simulink model "Purdue_Sim_Fast"  (R2018b)
settings: Solver=VariableStepAuto  StartTime=0.0  StopTime=300  RelTol=1e-3
values from neighbouring files (symbols this model uses):
  burn_time = (200000+Impulse_Savings)/Thrust    [One_Run.m]    (also in Purdue_Setup.m = 40; Setup.m = 42; Test_Runs.m = 40; Test_Runs_Arthur_Function.m = 42.7553241067)
  data = [Mass_b Mass_c]    [Boattail.m]    (also in One_Run.m = load('aerodata.csv'); Purdue_Setup.m = load('aerodata.csv'); Setup.m = load('aerodata.csv'); Test_Runs.m = load('aerodata.csv'))
  diameter_ft = diameter / 12    (= 1.5)    [One_Run.m]    (also in Purdue_Setup.m; Setup.m = 0.535416666667; Test_Runs.m; Test_Runs_Arthur_Function.m)
  dry_mass_slugs = dry_mass / 32.2    [One_Run.m]    (also in Purdue_Setup.m = 12.4223602484; Setup.m = 1.28260869565; Test_Runs.m; Test_Runs_Arthur_Function.m)
  m_dot_slugs = m_dot / 32.2    (= 0.585403726708)    [One_Run.m]    (also in Purdue_Setup.m = -0.621118012422; Setup.m = 0.0567139899438; Test_Runs.m = -0.621118012422; Test_Runs_Arthur_Function.m = -0.62217941157)
  wet_mass_slugs = wet_mass / 32.2    (= 40.8444099379)    [One_Run.m]    (also in Purdue_Setup.m = 37.2670807453; Setup.m = 3.66459627329; Test_Runs.m = wet_mass / 32.2; Test_Runs_Arthur_Function.m = wet_mass / 32.2)
undefined symbols (not defined in the file or in its folder): Thurst
libraries: aerolibasang x2, aerolibconvert2 x2, shared6dof x1, aerolibadyn x1, aerolibatmos2 x1, simulink x1, vrlib x1
settings Model: PacingRate=1000  Creator=jbartkie  LastModifiedBy=bartk
settings DebuggingCC: LibraryContextMissingDiagnostic=none  UnderSpecifiedDimensionMsg=warning
settings SFSimCC: SimUseLocalCustomCode=off
settings RTWCC: RTWUseLocalCustomCode=off

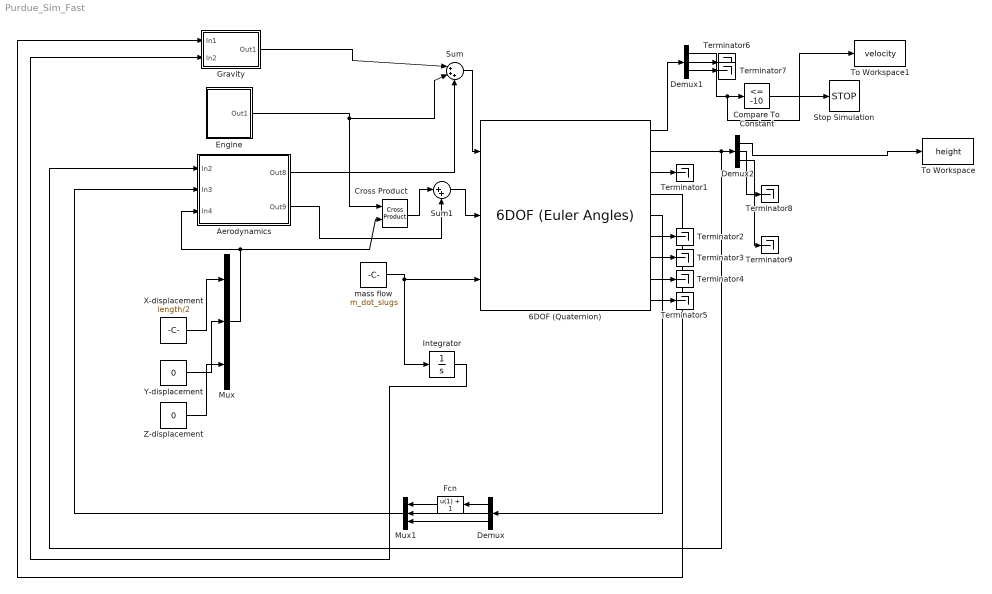
== system Purdue_Sim_Fast ==
  6DOF (Quaternion) : shared6dof/6DOF (Euler Angles)  units=English (Velocity in ft/s)  mtype=Simple Variable  rep=Quaternion  xme_0=[0 0 0]  Vm_0=[0 0 0]  eul_0=[0 0 0]  pm_0=[0 0 0]  mass_0=wet_mass_slugs  mass_e=dry_mass_slugs  mass_f=wet_mass_slugs  inertia=eye(3)  inertia_e=I_wet  inertia_f=I_dry  k_quat=1.0  vre_flag=off  abi_flag=off  aMode=0  xme_statename=''  Vm_statename=''  eul_statename=''  quat_statename=''  pm_statename=''  mass_statename=''
      settings: SourceProductBaseCode=AE
  "Aerodynamics " : Subsystem
  Compare To Constant : simulink/Logic and Bit Operations/Compare To Constant  relop=<=  const=-10  OutDataTypeStr=boolean
  Cross Product : vrlib/Utilities/Cross Product
      settings: SourceProductBaseCode=VR
  Demux : Demux  Outputs=3
  Demux1 : Demux  Outputs=3
  Demux2 : Demux  Outputs=3
  "Engine " : Subsystem
  Fcn : Fcn  Expr=u(1) + 1
  Gravity : Subsystem
  Integrator : Integrator  InitialCondition=wet_mass_slugs  LimitOutput=on  LowerSaturationLimit=dry_mass_slugs
  Mux : Mux  Inputs=3
  Mux1 : Mux  Inputs=3
  Stop Simulation : Stop
  Sum : Sum  Inputs=|+++
  Sum1 : Sum  Inputs=|++
  Terminator{1..9} (9 alike) : Terminator
  To Workspace : ToWorkspace  VariableName=height  SaveFormat=Timeseries  SampleTime=-1
  To Workspace1 : ToWorkspace  VariableName=velocity  SaveFormat=Timeseries  SampleTime=-1
  X-displacement : Constant  Value=length/2
  Y-displacement : Constant  Value=0
  Z-displacement : Constant  Value=0
  mass flow : Constant  Value=m_dot_slugs
  wires:
  Z-displacement/1 -> Mux/3
  X-displacement/1 -> Mux/1
  Y-displacement/1 -> Mux/2
  "Engine "/1(Out1) -> Cross Product/1, Sum/2
  Sum/1 -> 6DOF (Quaternion)/1
  Gravity/1(Out1) -> Sum/1
  Integrator/1 -> Gravity/2(In2)
  mass flow/1 -> Integrator/1, 6DOF (Quaternion)/3
  6DOF (Quaternion)/4 -> Gravity/1(In1)
  Sum1/1 -> 6DOF (Quaternion)/2
  Cross Product/1 -> Sum1/1
  Mux/1 -> Cross Product/2, "Aerodynamics "/3(In4)
  "Aerodynamics "/1(Out8) -> Sum/3
  "Aerodynamics "/2(Out9) -> Sum1/2
  6DOF (Quaternion)/5 -> Demux/1
  Demux/2 -> Mux1/2
  Demux/3 -> Mux1/3
  Demux/1 -> Fcn/1
  Fcn/1 -> Mux1/1
  Mux1/1 -> "Aerodynamics "/2(In3)
  6DOF (Quaternion)/1 -> Demux1/1
  6DOF (Quaternion)/3 -> Terminator1/1
  6DOF (Quaternion)/6 -> Terminator2/1
  6DOF (Quaternion)/7 -> Terminator3/1
  6DOF (Quaternion)/8 -> Terminator4/1
  6DOF (Quaternion)/9 -> Terminator5/1
  6DOF (Quaternion)/2 -> Demux2/1, "Aerodynamics "/1(In2)
  Demux1/1 -> To Workspace1/1, Compare To Constant/1
  Compare To Constant/1 -> Stop Simulation/1
  Demux1/2 -> Terminator6/1
  Demux1/3 -> Terminator7/1
  Demux2/1 -> To Workspace/1
  Demux2/2 -> Terminator8/1
  Demux2/3 -> Terminator9/1

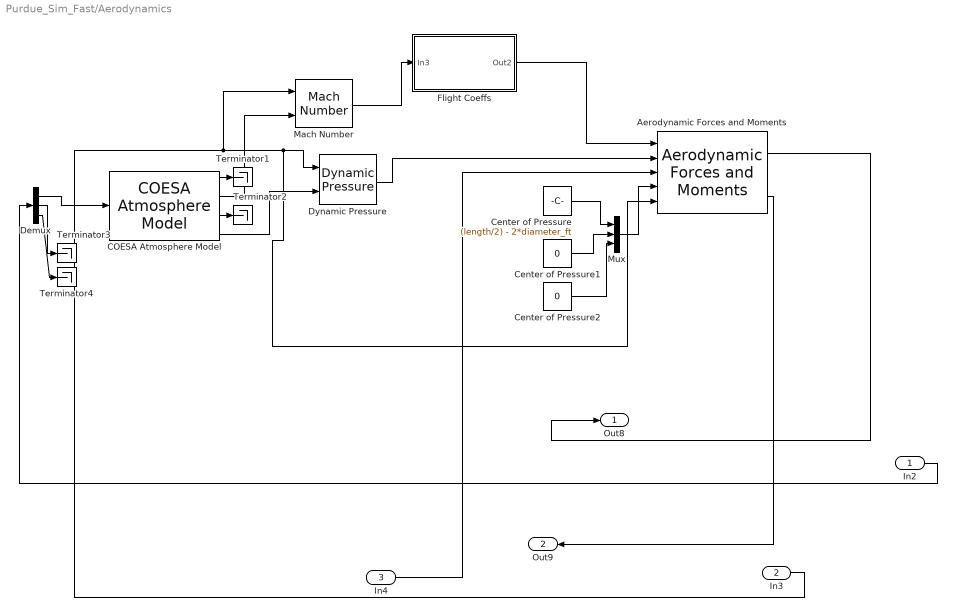
== system Purdue_Sim_Fast/Aerodynamics  ==
  In2 : Inport
  In3 : Inport  Port=2
  In4 : Inport  Port=3
  "Aerodynamic Forces and Moments " : aerolibadyn/Aerodynamic Forces and Moments   inputAxes=Wind  outputForceAxes=Body  outputMomentAxes=Body  S=(diameter_ft/2)^2 * pi  b=diameter_ft  cbar=length
      settings: SourceProductName=Aerospace Blockset
  COESA Atmosphere Model : aerolibatmos2/COESA Atmosphere Model  units=English (Velocity in ft/s)  spec=1976 COESA-extended U.S. Standard Atmosphere  model=Profile  profile_var=High temperature  profile_percent=1%  profile_alt=5 km (16404 ft)  envelope_var=High temperature  envelope_percent=1%  action=Warning
  Center of Pressure : Constant  Value=(length/2) - 2*diameter_ft
  Center of Pressure1 : Constant  Value=0
  Center of Pressure2 : Constant  Value=0
  Demux : Demux  Outputs=3
  Dynamic Pressure : aerolibasang/Dynamic Pressure
  Flight Coeffs : Subsystem
  Mach Number : aerolibasang/Mach Number
      settings: SourceProductName=Aerospace Blockset  SourceProductBaseCode=AE
  Mux : Mux  Inputs=3
  Terminator{1..4} (4 alike) : Terminator
  Out8 : Outport
  Out9 : Outport  Port=2
  wires:
  Dynamic Pressure/1 -> "Aerodynamic Forces and Moments "/2
  Demux/1 -> COESA Atmosphere Model/1
  In2/1 -> Demux/1
  In4/1 -> "Aerodynamic Forces and Moments "/3
  COESA Atmosphere Model/4 -> Dynamic Pressure/2
  COESA Atmosphere Model/2 -> Mach Number/2
  In3/1 -> Mach Number/1, "Aerodynamic Forces and Moments "/5, Dynamic Pressure/1
  "Aerodynamic Forces and Moments "/2 -> Out9/1
  Mach Number/1 -> Flight Coeffs/1(In3)
  Flight Coeffs/1(Out2) -> "Aerodynamic Forces and Moments "/1
  Mux/1 -> "Aerodynamic Forces and Moments "/4
  Center of Pressure/1 -> Mux/1
  Center of Pressure1/1 -> Mux/2
  Center of Pressure2/1 -> Mux/3
  "Aerodynamic Forces and Moments "/1 -> Out8/1
  COESA Atmosphere Model/1 -> Terminator1/1
  COESA Atmosphere Model/3 -> Terminator2/1
  Demux/2 -> Terminator3/1
  Demux/3 -> Terminator4/1

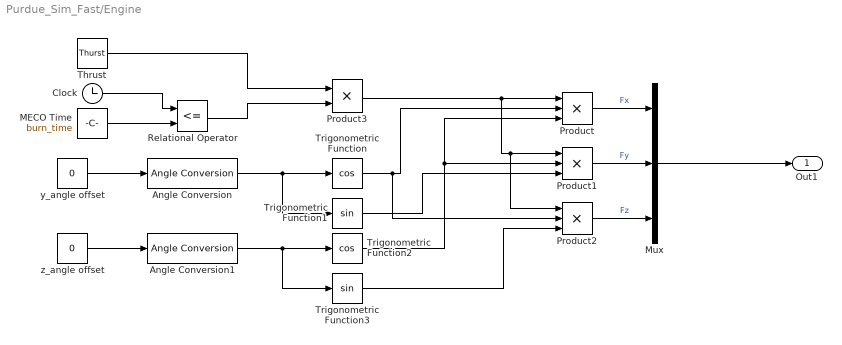
== system Purdue_Sim_Fast/Engine  ==
  Angle Conversion : aerolibconvert2/Angle Conversion  IU=deg  OU=rad
  Angle Conversion1 : aerolibconvert2/Angle Conversion  IU=deg  OU=rad
  Clock : Clock
  MECO Time : Constant  Value=burn_time
  Mux : Mux  Inputs=3
  Product : Product  Inputs=3
  Product1 : Product  Inputs=3
  Product2 : Product  Inputs=3
  Product3 : Product
  Relational Operator : RelationalOperator  Operator=<=  OutDataTypeStr=boolean  RndMeth=Simplest
  Thrust : Constant  Value=Thurst
  Trigonometric Function : Trigonometry  Operator=cos
  Trigonometric Function1 : Trigonometry
  Trigonometric Function2 : Trigonometry  Operator=cos
  Trigonometric Function3 : Trigonometry
  y_angle offset : Constant  Value=0
  z_angle offset : Constant  Value=0
  Out1 : Outport
  wires:
  Angle Conversion/1 -> Trigonometric Function1/1, Trigonometric Function/1
  Angle Conversion1/1 -> Trigonometric Function3/1, Trigonometric Function2/1
  Clock/1 -> Relational Operator/1
  MECO Time/1 -> Relational Operator/2
  Thrust/1 -> Product3/1
  Relational Operator/1 -> Product3/2
  Product/1 -> Mux/1  "Fx"
  Product1/1 -> Mux/2  "Fy"
  Product2/1 -> Mux/3  "Fz"
  Mux/1 -> Out1/1
  Product3/1 -> Product2/1, Product1/1, Product/1
  Trigonometric Function2/1 -> Product1/2, Product/3
  Trigonometric Function/1 -> Product2/2, Product/2
  Trigonometric Function1/1 -> Product1/3
  Trigonometric Function3/1 -> Product2/3
  y_angle offset/1 -> Angle Conversion/1
  z_angle offset/1 -> Angle Conversion1/1

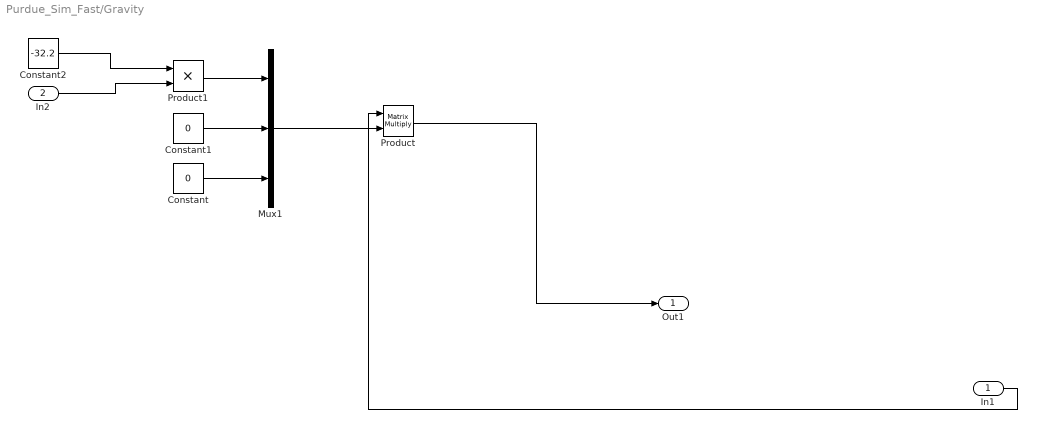
== system Purdue_Sim_Fast/Gravity ==
  In1 : Inport
  In2 : Inport  Port=2
  Constant : Constant  Value=0
  Constant1 : Constant  Value=0
  Constant2 : Constant  Value=-32.2
  Mux1 : Mux  Inputs=3
  Product : Product  Multiplication=Matrix(*)
  Product1 : Product
  Out1 : Outport
  wires:
  Mux1/1 -> Product/2
  Product/1 -> Out1/1
  In1/1 -> Product/1
  Constant1/1 -> Mux1/2
  Constant2/1 -> Product1/1
  In2/1 -> Product1/2
  Product1/1 -> Mux1/1
  Constant/1 -> Mux1/3

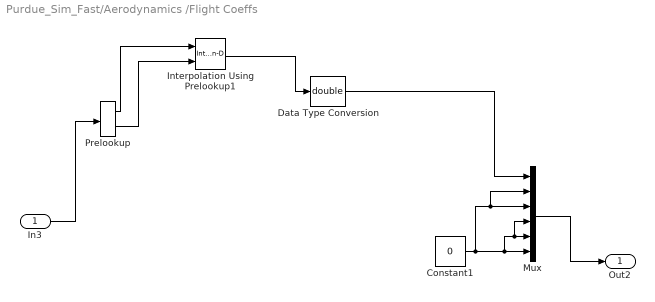
== system Purdue_Sim_Fast/Aerodynamics /Flight Coeffs ==
  In3 : Inport
  Constant1 : Constant  Value=0
  Data Type Conversion : DataTypeConversion  OutDataTypeStr=double
  Interpolation Using Prelookup1 : Interpolation_n-D  NumberOfTableDimensions=1  Table=data(:,3)  InternalRulePriority=Speed
      settings: InputPortMap=u0,u1
  Mux : Mux  Inputs=6
  Prelookup : PreLookup  BreakpointsData=data(:,1)  ExtrapMethod=Linear
  Out2 : Outport
  wires:
  Prelookup/2 -> Interpolation Using Prelookup1/2
  Constant1/1 -> Mux/2, Mux/3, Mux/4, Mux/5, Mux/6
  Interpolation Using Prelookup1/1 -> Data Type Conversion/1
  In3/1 -> Prelookup/1
  Mux/1 -> Out2/1
  Data Type Conversion/1 -> Mux/1
  Prelookup/1 -> Interpolation Using Prelookup1/1
